simulink model "Flight_Control"  (R2024b)
settings: configuration reference "csSingleInstance" (kept outside this file)
libraries: simulink x1
Description:
  | This is the top-level model of the helicopter flight control software.
settings Model: DataDictionary=DD_Flight_Control.sldd  EnableAccessToBaseWorkspace=off  Creator=The MathWorks, Inc.  LastModifiedBy=The MathWorks, Inc.
settings ConfigSetRef: SourceName=csSingleInstance

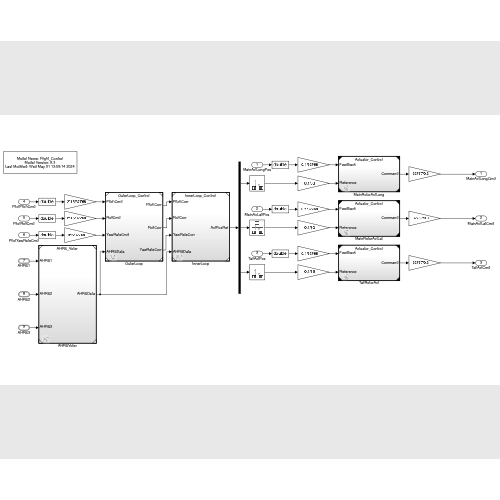
[thumbnail: Simulink's stored preview of the top-level diagram]
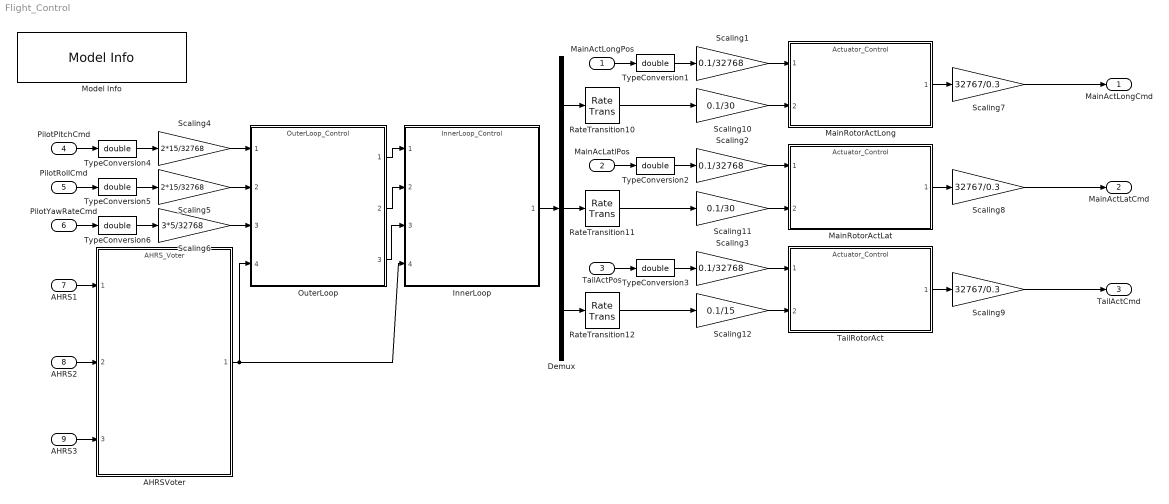
== system Flight_Control ==
  MainActLongPos : Inport  OutMin=-32768  OutMax=32767  OutDataTypeStr=int16  PortDimensions=1  SampleTime=0.001
  MainAcLatlPos : Inport  Port=2  OutMin=-32768  OutMax=32767  OutDataTypeStr=int16  PortDimensions=1  SampleTime=0.001
  TailActPos : Inport  Port=3  OutMin=-32768  OutMax=32767  OutDataTypeStr=int16  PortDimensions=1  SampleTime=0.001
  PilotPitchCmd : Inport  Port=4  OutMin=-32768  OutMax=32767  OutDataTypeStr=int16  PortDimensions=1  SampleTime=0.01
  PilotRollCmd : Inport  Port=5  OutMin=-32768  OutMax=32767  OutDataTypeStr=int16  PortDimensions=1  SampleTime=0.01
  PilotYawRateCmd : Inport  Port=6  OutMin=-32768  OutMax=32767  OutDataTypeStr=int16  PortDimensions=1  SampleTime=0.01
  AHRS1 : Inport  Port=7  OutDataTypeStr=Bus: AHRS_Bus  PortDimensions=1  SampleTime=0.01  BusOutputAsStruct=on
  AHRS2 : Inport  Port=8  OutDataTypeStr=Bus: AHRS_Bus  PortDimensions=1  SampleTime=0.01  BusOutputAsStruct=on
  AHRS3 : Inport  Port=9  OutDataTypeStr=Bus: AHRS_Bus  PortDimensions=1  SampleTime=0.01  BusOutputAsStruct=on
  AHRSVoter : ModelReference  ModelNameDialog=AHRS_Voter  SimulationMode=Normal  ModelReferenceVersion=8.0
  Demux : Demux  Outputs=3
  InnerLoop : ModelReference  ModelNameDialog=InnerLoop_Control  SimulationMode=Normal  ModelReferenceVersion=10.0
  MainRotorActLat : ModelReference  ModelNameDialog=Actuator_Control  UsingDefaultArgumentValue=0,0,0,0  ModelReferenceVersion=9.0  Kp=0.3  Ki=0.12  Kd=0.02  N=0.008
  MainRotorActLong : ModelReference  ModelNameDialog=Actuator_Control  UsingDefaultArgumentValue=0,0,0,0  ModelReferenceVersion=9.0  Kp=0.3  Ki=0.12  Kd=0.02  N=0.008
  Model Info : simulink/Model-Wide Utilities/Model Info  Frame=on  DisplayStringWithTags=|  HorizontalTextAlignment=Center  LeftAlignmentValue=0.5
      | Model Name: %<ModelName>
      | Model Version: %<ModelVersion>
      | Last Modified: %<LastModificationDate>
  OuterLoop : ModelReference  ModelNameDialog=OuterLoop_Control  SimulationMode=Normal  ModelReferenceVersion=8.0
  RateTransition10 : RateTransition  OutPortSampleTime=0.001
  RateTransition11 : RateTransition  OutPortSampleTime=0.001
  RateTransition12 : RateTransition  OutPortSampleTime=0.001
  Scaling1 : Gain  Gain=0.1/32768
  Scaling10 : Gain  Gain=0.1/30
  Scaling11 : Gain  Gain=0.1/30
  Scaling12 : Gain  Gain=0.1/15
  Scaling2 : Gain  Gain=0.1/32768
  Scaling3 : Gain  Gain=0.1/32768
  Scaling4 : Gain  Gain=2*15/32768
  Scaling5 : Gain  Gain=2*15/32768
  Scaling6 : Gain  Gain=3*5/32768
  Scaling7 : Gain  Gain=32767/0.3  SaturateOnIntegerOverflow=on  OutDataTypeStr=Inherit: Same as input
  Scaling8 : Gain  Gain=32767/0.3  SaturateOnIntegerOverflow=on  OutDataTypeStr=Inherit: Same as input
  Scaling9 : Gain  Gain=32767/0.3  SaturateOnIntegerOverflow=on  OutDataTypeStr=Inherit: Same as input
  TailRotorAct : ModelReference  ModelNameDialog=Actuator_Control  UsingDefaultArgumentValue=0,0,0,0  ModelReferenceVersion=9.0  Kp=0.3  Ki=0.12  Kd=0.02  N=0.008
  TypeConversion{1..6} (6 alike) : DataTypeConversion  OutDataTypeStr=double  SaturateOnIntegerOverflow=off  RndMeth=Floor
  MainActLongCmd : Outport  OutDataTypeStr=double  VectorParamsAs1DForOutWhenUnconnected=off
  MainActLatCmd : Outport  Port=2  OutDataTypeStr=double  VectorParamsAs1DForOutWhenUnconnected=off
  TailActCmd : Outport  Port=3  OutDataTypeStr=double  VectorParamsAs1DForOutWhenUnconnected=off
  wires:
  MainRotorActLong/1 -> Scaling7/1
  MainRotorActLat/1 -> Scaling8/1
  TailRotorAct/1 -> Scaling9/1
  RateTransition10/1 -> Scaling10/1
  RateTransition11/1 -> Scaling11/1
  RateTransition12/1 -> Scaling12/1
  AHRS2/1 -> AHRSVoter/2
  AHRS3/1 -> AHRSVoter/3
  Demux/1 -> RateTransition10/1
  Demux/2 -> RateTransition11/1
  Demux/3 -> RateTransition12/1
  InnerLoop/1 -> Demux/1
  AHRS1/1 -> AHRSVoter/1
  TypeConversion4/1 -> Scaling4/1
  PilotPitchCmd/1 -> TypeConversion4/1
  TypeConversion5/1 -> Scaling5/1
  PilotRollCmd/1 -> TypeConversion5/1
  PilotYawRateCmd/1 -> TypeConversion6/1
  TypeConversion6/1 -> Scaling6/1
  TypeConversion1/1 -> Scaling1/1
  MainActLongPos/1 -> TypeConversion1/1
  Scaling1/1 -> MainRotorActLong/1
  TypeConversion2/1 -> Scaling2/1
  TypeConversion3/1 -> Scaling3/1
  MainAcLatlPos/1 -> TypeConversion2/1
  Scaling2/1 -> MainRotorActLat/1
  TailActPos/1 -> TypeConversion3/1
  Scaling3/1 -> TailRotorAct/1
  Scaling7/1 -> MainActLongCmd/1
  Scaling8/1 -> MainActLatCmd/1
  Scaling9/1 -> TailActCmd/1
  Scaling4/1 -> OuterLoop/1
  Scaling5/1 -> OuterLoop/2
  Scaling6/1 -> OuterLoop/3
  OuterLoop/1 -> InnerLoop/1
  OuterLoop/2 -> InnerLoop/2
  OuterLoop/3 -> InnerLoop/3
  AHRSVoter/1 -> InnerLoop/4, OuterLoop/4
  Scaling10/1 -> MainRotorActLong/2
  Scaling11/1 -> MainRotorActLat/2
  Scaling12/1 -> TailRotorAct/2
